simulink model "Lab8"  (R2018b)
settings: Solver=VariableStepAuto  StartTime=0.0  StopTime=10.0  RelTol=1e-3
settings Model: Creator=Gość  LastModifiedBy=Gość

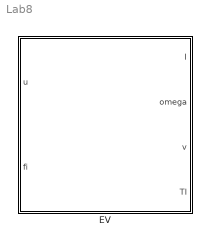
== system Lab8 ==
  EV : Subsystem

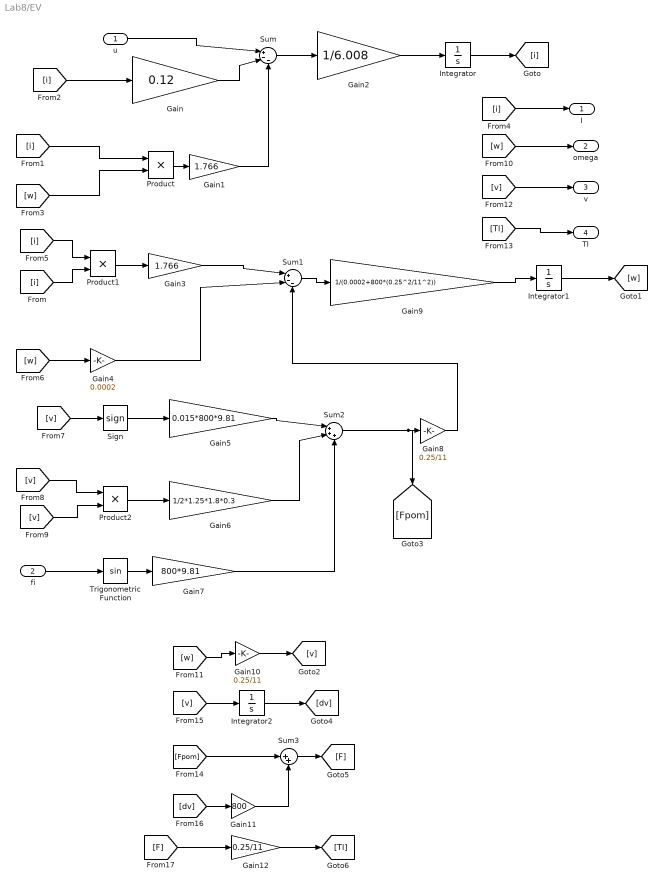
== system Lab8/EV ==
  u : Inport
  fi : Inport  Port=2
  Gain : Gain  Gain=0.12
  Gain1 : Gain  Gain=1.766
  Gain10 : Gain  Gain=0.25/11
  Gain11 : Gain  Gain=800
  Gain12 : Gain  Gain=0.25/11
  Gain2 : Gain  Gain=1/6.008
  Gain3 : Gain  Gain=1.766
  Gain4 : Gain  Gain=0.0002
  Gain5 : Gain  Gain=0.015*800*9.81
  Gain6 : Gain  Gain=1/2*1.25*1.8*0.3
  Gain7 : Gain  Gain=800*9.81
  Gain8 : Gain  Gain=0.25/11
  Gain9 : Gain  Gain=1/(0.0002+800*(0.25^2/11^2))
  Integrator : Integrator
  Integrator1 : Integrator
  Integrator2 : Integrator
  Product : Product
  Product1 : Product
  Product2 : Product
  Sign : Signum
  Sum : Sum  Inputs=|+--
  Sum1 : Sum  Inputs=|+--
  Sum2 : Sum  Inputs=|+++
  Sum3 : Sum  Inputs=|++
  Trigonometric Function : Trigonometry
  I : Outport
  "omega " : Outport  Port=2
  v : Outport  Port=3
  TI : Outport  Port=4
  wires:
  [i] -> Product/1
  Sum/1 -> Gain2/1
  u/1 -> Sum/1
  Gain/1 -> Sum/2
  Gain1/1 -> Sum/3
  Integrator/1 -> [i]
  Product/1 -> Gain1/1
  [w] -> Product/2
  [i] -> Gain/1
  Gain2/1 -> Integrator/1
  [i] -> I/1
  [i] -> Product1/1
  [i] -> Product1/2
  Product1/1 -> Gain3/1
  Gain3/1 -> Sum1/1
  [w] -> Gain4/1
  Gain4/1 -> Sum1/2
  [v] -> Sign/1
  Sign/1 -> Gain5/1
  Gain5/1 -> Sum2/1
  [v] -> Product2/1
  [v] -> Product2/2
  Product2/1 -> Gain6/1
  Gain6/1 -> Sum2/2
  Trigonometric Function/1 -> Gain7/1
  Gain7/1 -> Sum2/3
  Sum2/1 -> [Fpom], Gain8/1
  Gain8/1 -> Sum1/3
  Sum1/1 -> Gain9/1
  Gain9/1 -> Integrator1/1
  Integrator1/1 -> [w]
  [w] -> Gain10/1
  Gain10/1 -> [v]
  fi/1 -> Trigonometric Function/1
  [w] -> "omega "/1
  [v] -> v/1
  [v] -> Integrator2/1
  Integrator2/1 -> [dv]
  [dv] -> Gain11/1
  Gain11/1 -> Sum3/2
  [Fpom] -> Sum3/1
  Sum3/1 -> [F]
  [F] -> Gain12/1
  Gain12/1 -> [Tl]
  [Tl] -> TI/1
